simulink model "Simulink_Control_BlueROV_Modo_Deslizante"  (R2019a)
settings: Solver=VariableStepAuto  StartTime=0.0  StopTime=100*3  RelTol=1e-3
values from neighbouring files (symbols this model uses):
  a0 = 50    [Control_BlueROV_Modo_Deslizante.m]
  a1 = 1    [Control_BlueROV_Modo_Deslizante.m]
  B = 78.38    [Control_BlueROV_Modo_Deslizante.m]
  eta = 1    [Control_BlueROV_Modo_Deslizante.m]
  Ix = 0.16    [Control_BlueROV_Modo_Deslizante.m]
  Ixy = 0    [Control_BlueROV_Modo_Deslizante.m]
  Ixz = 0    [Control_BlueROV_Modo_Deslizante.m]
  Iy = 0.16    [Control_BlueROV_Modo_Deslizante.m]
  Iyz = 0    [Control_BlueROV_Modo_Deslizante.m]
  Iz = 0.16    [Control_BlueROV_Modo_Deslizante.m]
  Kp = -0.07    [Control_BlueROV_Modo_Deslizante.m]
  Kpdot = -0.12    [Control_BlueROV_Modo_Deslizante.m]
  Kpp = -1.55    [Control_BlueROV_Modo_Deslizante.m]
  m = 7.31    [Control_BlueROV_Modo_Deslizante.m]
  M = Mrb+Ma    [Control_BlueROV_Modo_Deslizante.m]
  Minv = inv(M)    [Control_BlueROV_Modo_Deslizante.m]
  Mq = -0.07    [Control_BlueROV_Modo_Deslizante.m]
  Mqdot = -0.12    [Control_BlueROV_Modo_Deslizante.m]
  Mqq = -1.55    [Control_BlueROV_Modo_Deslizante.m]
  Nr = -0.07    [Control_BlueROV_Modo_Deslizante.m]
  Nrdot = -0.12    [Control_BlueROV_Modo_Deslizante.m]
  Nrr = -1.55    [Control_BlueROV_Modo_Deslizante.m]
  W = 71.71    [Control_BlueROV_Modo_Deslizante.m]
  xb = 0    [Control_BlueROV_Modo_Deslizante.m]
  xg = 0    [Control_BlueROV_Modo_Deslizante.m]
  Xu = -4.03    [Control_BlueROV_Modo_Deslizante.m]
  Xudot = -5.5    [Control_BlueROV_Modo_Deslizante.m]
  Xuu = -18.18    [Control_BlueROV_Modo_Deslizante.m]
  yb = 0    [Control_BlueROV_Modo_Deslizante.m]
  yg = 0    [Control_BlueROV_Modo_Deslizante.m]
  Yv = -6.22    [Control_BlueROV_Modo_Deslizante.m]
  Yvdot = -12.7    [Control_BlueROV_Modo_Deslizante.m]
  Yvv = -21.66    [Control_BlueROV_Modo_Deslizante.m]
  zb = 0.00019    [Control_BlueROV_Modo_Deslizante.m]
  zg = 0    [Control_BlueROV_Modo_Deslizante.m]
  Zw = -5.18    [Control_BlueROV_Modo_Deslizante.m]
  Zwdot = -14.57    [Control_BlueROV_Modo_Deslizante.m]
  Zww = -36.99    [Control_BlueROV_Modo_Deslizante.m]
(part 1 of 2)
settings Model: Creator=andres lopez  LastModifiedBy=andres lopez

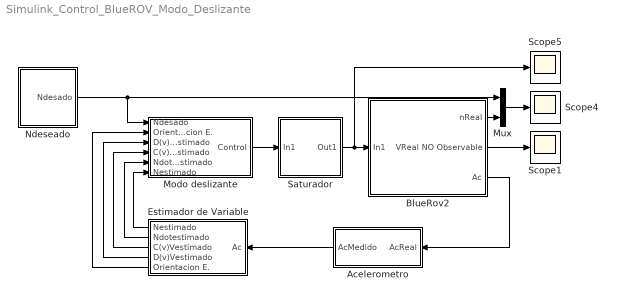
== system Simulink_Control_BlueROV_Modo_Deslizante ==
  Acelerometro : Subsystem
  BlueRov2 : Subsystem
  Estimador de Variable : Subsystem
  Modo deslizante : Subsystem
  Mux : Mux  Inputs=2
  Ndeseado : Subsystem
  Saturador : Subsystem
  Scope1 : Scope
  Scope4 : Scope
  Scope5 : Scope
  wires:
  BlueRov2/2("VReal NO Observable ") -> Scope1/1
  BlueRov2/1(nReal) -> Mux/2
  Ndeseado/1(Ndesado) -> Modo deslizante/1(Ndesado), Mux/1
  Mux/1 -> Scope4/1
  Saturador/1(Out1) -> Scope5/1, BlueRov2/1(In1)
  Modo deslizante/1(Control) -> Saturador/1(In1)
  Estimador de Variable/1(Nestimado) -> Modo deslizante/6(Nestimado)
  Estimador de Variable/2(Ndotestimado) -> Modo deslizante/5(Ndotestimado)
  Estimador de Variable/3(C(v)Vestimado) -> Modo deslizante/4(C(v)Vestimado)
  Estimador de Variable/4(D(v)Vestimado) -> Modo deslizante/3("D(v)Vestimado ")
  Estimador de Variable/5(Orientacion E.) -> Modo deslizante/2(Orientacion E.)
  BlueRov2/3(Ac) -> Acelerometro/1(AcReal)
  Acelerometro/1(AcMedido) -> Estimador de Variable/1(Ac)

== system Simulink_Control_BlueROV_Modo_Deslizante/Acelerometro ==
  AcReal : Inport
  Gain : Gain
  AcMedido : Outport
  wires:
  Gain/1 -> AcMedido/1
  AcReal/1 -> Gain/1

== system Simulink_Control_BlueROV_Modo_Deslizante/BlueRov2 ==
  In1 : Inport
  Add : Sum  Inputs=+---+
  C(v) : Subsystem
  D(v) : Subsystem
  Integrator : Integrator
  Integrator1 : Integrator
  J(n) : Subsystem
  "Perturbacion " : Step  Time=250  After=[2;-2;-3;0;0;0]  SampleTime=0
  g(n) : Subsystem
  inv(Matriz de masa Inercial) : Subsystem
  nReal : Outport
  "VReal NO Observable " : Outport  Port=2
  Ac : Outport  Port=3
  wires:
  In1/1 -> Add/1
  Add/1 -> inv(Matriz de masa Inercial)/1(Inercia)
  J(n)/1(Out1) -> Integrator1/1
  inv(Matriz de masa Inercial)/1(Aceleracion) -> Ac/1, Integrator/1
  g(n)/1(Out1) -> Add/2
  D(v)/1(Out1) -> Add/3
  Integrator1/1 -> g(n)/1(In1), J(n)/2(In2), nReal/1
  Integrator/1 -> "VReal NO Observable "/1, D(v)/1(In1), C(v)/1(In1), J(n)/1(In1)
  C(v)/1(Out1) -> Add/4
  "Perturbacion "/1 -> Add/5

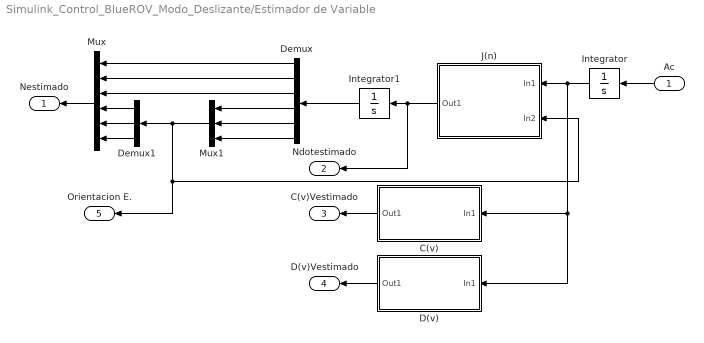
== system Simulink_Control_BlueROV_Modo_Deslizante/Estimador de Variable ==
  Ac : Inport
  C(v) : Subsystem
  D(v) : Subsystem
  Demux : Demux  Outputs=6
  Demux1 : Demux  Outputs=3
  Integrator : Integrator
  Integrator1 : Integrator
  J(n) : Subsystem
  Mux : Mux  Inputs=6
  Mux1 : Mux  Inputs=3
  Nestimado : Outport
  Ndotestimado : Outport  Port=2
  C(v)Vestimado : Outport  Port=3
  D(v)Vestimado : Outport  Port=4
  Orientacion E. : Outport  Port=5
  wires:
  Ac/1 -> Integrator/1
  Integrator/1 -> D(v)/1(In1), C(v)/1(In1), J(n)/1(In1)
  J(n)/1(Out1) -> Ndotestimado/1, Integrator1/1
  C(v)/1(Out1) -> C(v)Vestimado/1
  D(v)/1(Out1) -> D(v)Vestimado/1
  Integrator1/1 -> Demux/1
  Demux/1 -> Mux/1
  Demux/2 -> Mux/2
  Demux1/2 -> Mux/5
  Demux1/1 -> Mux/4
  Demux1/3 -> Mux/6
  Mux/1 -> Nestimado/1
  Demux/3 -> Mux/3
  Mux1/1 -> Orientacion E./1, J(n)/2(In2), Demux1/1
  Demux/4 -> Mux1/1
  Demux/5 -> Mux1/2
  Demux/6 -> Mux1/3

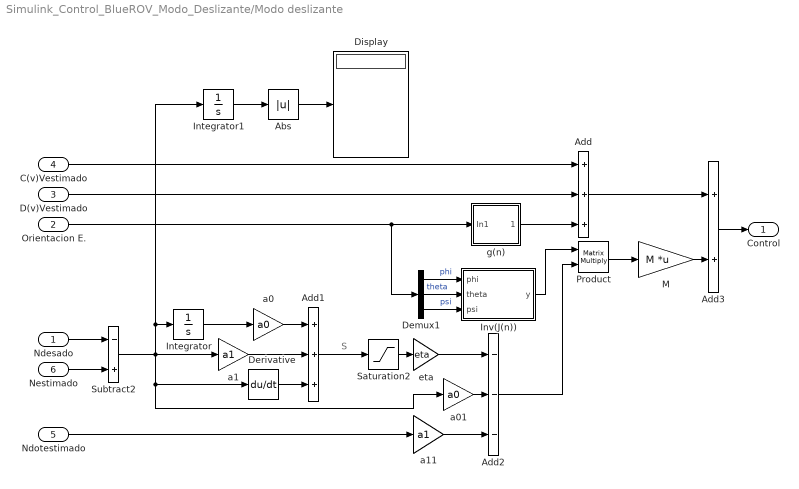
== system Simulink_Control_BlueROV_Modo_Deslizante/Modo deslizante ==
  note: S
  Ndesado : Inport
  Orientacion E. : Inport  Port=2
  "D(v)Vestimado " : Inport  Port=3
  C(v)Vestimado : Inport  Port=4
  Ndotestimado : Inport  Port=5
  Nestimado : Inport  Port=6
  Abs : Abs
  Add : Sum  Inputs=+++
  Add1 : Sum  Inputs=+++
  Add2 : Sum  Inputs=---
  Add3 : Sum
  Demux1 : Demux  Outputs=3
  Derivative : Derivative
  Display : Display
  Integrator : Integrator
  Integrator1 : Integrator
  Inv(J(n)) : MATLAB Function  TreatAsAtomicUnit=on
  M : Gain  Gain=M  Multiplication=Matrix(K*u) (u vector)
  Product : Product  Multiplication=Matrix(*)
  Saturation2 : Saturate  UpperLimit=1  LowerLimit=-1
  Subtract2 : Sum  Inputs=-+
  "a0 " : Gain  Gain=a0
  a01 : Gain  Gain=a0
  a1 : Gain  Gain=a1
  a11 : Gain  Gain=a1
  eta : Gain  Gain=eta
  g(n) : Subsystem
  Control : Outport
  wires:
  Ndotestimado/1 -> a11/1
  Orientacion E./1 -> Demux1/1, g(n)/1(In1)
  a11/1 -> Add2/3
  eta/1 -> Add2/1
  Demux1/1 -> Inv(J(n))/1(phi)  "phi"
  Demux1/3 -> Inv(J(n))/3(psi)  "psi"
  Add2/1 -> Product/2
  Saturation2/1 -> eta/1
  Product/1 -> M/1
  Inv(J(n))/1(y) -> Product/1
  a01/1 -> Add2/2
  Demux1/2 -> Inv(J(n))/2(theta)  "theta"
  Integrator1/1 -> Abs/1
  Abs/1 -> Display/1
  Add3/1 -> Control/1
  M/1 -> Add3/2
  Add/1 -> Add3/1
  Nestimado/1 -> Subtract2/2
  Ndesado/1 -> Subtract2/1
  g(n)/1(Out1) -> Add/3
  "D(v)Vestimado "/1 -> Add/2
  C(v)Vestimado/1 -> Add/1
  Subtract2/1 -> Integrator1/1, Integrator/1, a1/1, Derivative/1, a01/1
  Add1/1 -> Saturation2/1
  Derivative/1 -> Add1/3
  "a0 "/1 -> Add1/1
  a1/1 -> Add1/2
  Integrator/1 -> "a0 "/1

== system Simulink_Control_BlueROV_Modo_Deslizante/Ndeseado ==
  Euler 1 : Constant  Value=[0;0;0]
  Mux2 : Mux
  Uniform Random Number4 : UniformRandomNumber  Minimum=-10  Maximum=10  Seed=2  SampleTime=100
  Uniform Random Number5 : UniformRandomNumber  Minimum=0  Maximum=10  Seed=1  SampleTime=100
  Uniform Random Number6 : UniformRandomNumber  Minimum=-10  Maximum=10  Seed=3  SampleTime=100
  Ndesado : Outport
  wires:
  Uniform Random Number4/1 -> Mux2/2
  Uniform Random Number5/1 -> Mux2/3
  Euler 1/1 -> Mux2/4
  Mux2/1 -> Ndesado/1
  Uniform Random Number6/1 -> Mux2/1

== system Simulink_Control_BlueROV_Modo_Deslizante/Saturador ==
  In1 : Inport
  Demux3 : Demux  Outputs=6
  Mux1 : Mux  Inputs=3
  Mux2 : Mux
  Saturation : Saturate  UpperLimit=6.5  LowerLimit=-6.5
  Saturation1 : Saturate  UpperLimit=7.5  LowerLimit=-7.5
  Saturation2 : Saturate  UpperLimit=11  LowerLimit=4
  Saturation3 : Saturate  UpperLimit=3  LowerLimit=-3
  Out1 : Outport
  wires:
  Demux3/1 -> Saturation/1
  Saturation2/1 -> Mux2/3
  Saturation/1 -> Mux2/1
  Saturation3/1 -> Mux2/4
  Saturation1/1 -> Mux2/2
  Demux3/3 -> Saturation2/1
  Mux1/1 -> Saturation3/1
  Demux3/6 -> Mux1/3
  Demux3/2 -> Saturation1/1
  Demux3/5 -> Mux1/2
  Demux3/4 -> Mux1/1
  Mux2/1 -> Out1/1
  In1/1 -> Demux3/1

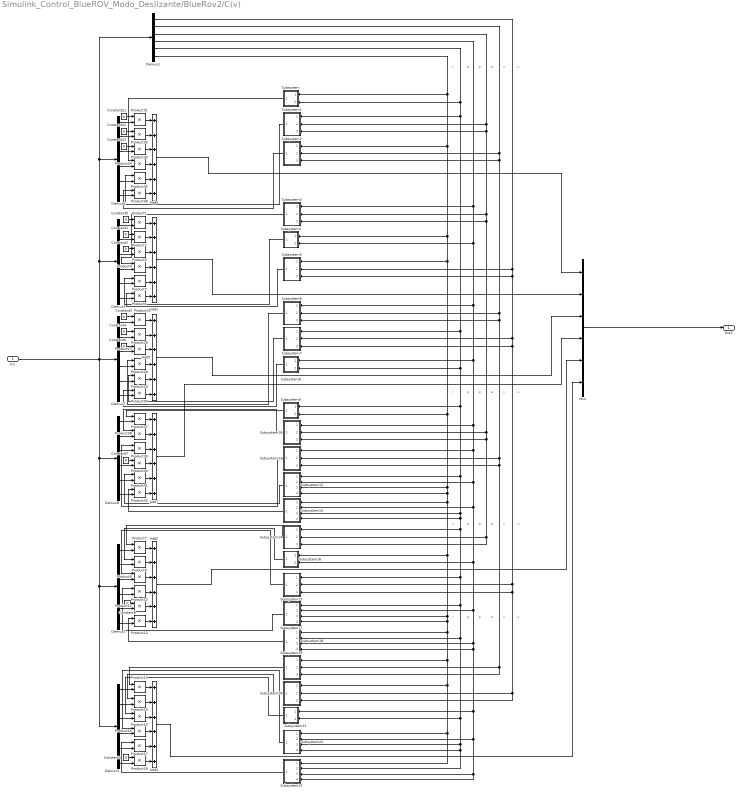
== system Simulink_Control_BlueROV_Modo_Deslizante/BlueRov2/C(v) ==
  note: u
  note: v
  note: w
  note: p
  note: q
  note: r
  note: v
  note: p
  note: u
  note: w
  note: q
  note: r
  note: v
  note: r
  note: w
  note: u
  note: q
  note: p
  note: v
  note: r
  note: w
  note: u
  note: q
  note: p
  In1 : Inport
  Add{1..3,5..7} (6 alike) : Sum  Inputs=++++++
  Constant{1..9,21..23} (12 alike) : Constant  Value=0
  Demux{1..3,5..8} (7 alike) : Demux  Outputs=6
  Mux : Mux  Inputs=6
  Product{1..18,25..42} (36 alike) : Product
  Subsystem : Subsystem
  Subsystem1 : Subsystem
  Subsystem10 : Subsystem
  Subsystem11 : Subsystem
  Subsystem12 : Subsystem
  Subsystem13 : Subsystem
  Subsystem14 : Subsystem
  Subsystem15 : Subsystem
  Subsystem16 : Subsystem
  Subsystem17 : Subsystem
  Subsystem18 : Subsystem
  Subsystem19 : Subsystem
  Subsystem2 : Subsystem
  Subsystem20 : Subsystem
  Subsystem21 : Subsystem
  Subsystem22 : Subsystem
  Subsystem23 : Subsystem
  Subsystem3 : Subsystem
  Subsystem4 : Subsystem
  Subsystem5 : Subsystem
  Subsystem6 : Subsystem
  Subsystem7 : Subsystem
  Subsystem8 : Subsystem
  Subsystem9 : Subsystem
  Out1 : Outport
  wires:
  In1/1 -> Demux5/1, Demux6/1, Demux1/1, Demux7/1, Demux8/1, Demux3/1, Demux2/1
  Product39/1 -> Add7/3
  Demux8/2 -> Product38/2
  Product36/1 -> Add6/6
  Product31/1 -> Add6/1
  Product35/1 -> Add6/5
  Demux6/2 -> Product32/2
  Demux6/4 -> Product34/2
  Demux6/5 -> Product35/2
  Product33/1 -> Add6/3
  Demux6/3 -> Product33/2
  Product5/1 -> Add1/5
  Demux5/2 -> Product2/2
  Product32/1 -> Add6/2
  Product41/1 -> Add7/5
  Product34/1 -> Add6/4
  Product2/1 -> Add1/2
  Demux8/5 -> Product41/2
  Product1/1 -> Add1/1
  Product18/1 -> Add3/6
  Product3/1 -> Add1/3
  Demux8/3 -> Product39/2
  Product8/1 -> Add2/2
  Demux2/6 -> Product12/2
  Product4/1 -> Add1/4
  Product37/1 -> Add7/1
  Demux5/1 -> Product1/2
  Demux8/6 -> Product42/2
  Demux5/4 -> Product4/2
  Demux5/5 -> Product5/2
  Product17/1 -> Add3/5
  Demux5/3 -> Product3/2
  Demux6/1 -> Product31/2
  Product13/1 -> Add3/1
  Product14/1 -> Add3/2
  Product40/1 -> Add7/4
  Product15/1 -> Add3/3
  Demux8/4 -> Product40/2
  Demux7/2 -> Product26/2
  Product42/1 -> Add7/6
  Product12/1 -> Add2/6
  Product26/1 -> Add5/2
  Product6/1 -> Add1/6
  Demux6/6 -> Product36/2
  Demux5/6 -> Product6/2
  Product29/1 -> Add5/5
  Product28/1 -> Add5/4
  Demux7/3 -> Product27/2
  Product16/1 -> Add3/4
  Product10/1 -> Add2/4
  Demux7/5 -> Product29/2
  Product9/1 -> Add2/3
  Product38/1 -> Add7/2
  Demux2/4 -> Product10/2
  Demux2/2 -> Product8/2
  Demux8/1 -> Product37/2
  Demux2/5 -> Product11/2
  Product7/1 -> Add2/1
  Product11/1 -> Add2/5
  Mux/1 -> Out1/1
  Demux7/4 -> Product28/2
  Demux2/1 -> Product7/2
  Demux7/6 -> Product30/2
  Product25/1 -> Add5/1
  Product27/1 -> Add5/3
  Product30/1 -> Add5/6
  Demux7/1 -> Product25/2
  Demux2/3 -> Product9/2
  Constant21/1 -> Product31/1
  Constant22/1 -> Product32/1
  Constant23/1 -> Product33/1
  Demux3/6 -> Product18/2
  Demux3/5 -> Product17/2
  Demux3/4 -> Product16/2
  Demux3/3 -> Product15/2
  Demux3/2 -> Product14/2
  Demux3/1 -> Product13/2
  Constant5/1 -> Product1/1
  Constant1/1 -> Product2/1
  Constant2/1 -> Product3/1
  Constant3/1 -> Product25/1
  Constant4/1 -> Product26/1
  Constant6/1 -> Product27/1
  Constant7/1 -> Product40/1
  Constant8/1 -> Product11/1
  Constant9/1 -> Product18/1
  Demux1/1 -> Subsystem5/2(In2), Subsystem15/2(In2), Subsystem15/3(In3), Subsystem20/2(In2), Subsystem20/3(In3), Subsystem7/3(In3), Subsystem7/2(In2), Subsystem5/3(In3)
  Demux1/2 -> Subsystem11/3(In3), Subsystem19/2(In2), Subsystem19/3(In3), Subsystem11/2(In2), Subsystem6/3(In3), Subsystem6/2(In2), Subsystem2/3(In3), Subsystem2/2(In2)
  Demux1/3 -> Subsystem3/2(In2), Subsystem3/3(In3), Subsystem10/2(In2), Subsystem10/3(In3), Subsystem14/2(In2), Subsystem14/3(In3), Subsystem1/3(In3), Subsystem1/2(In2)
  Subsystem/1(Out1) -> Product34/1
  Subsystem1/1(Out1) -> Product35/1
  Subsystem2/1(Out1) -> Product36/1
  Add6/1 -> Mux/1
  Subsystem3/1(Out1) -> Product4/1
  Subsystem4/1(Out1) -> Product5/1
  Subsystem5/1(Out1) -> Product6/1
  Add1/1 -> Mux/2
  Subsystem6/1(Out1) -> Product28/1
  Subsystem7/1(Out1) -> Product29/1
  Subsystem8/1(Out1) -> Product30/1
  Add5/1 -> Mux/3
  Subsystem9/1(Out1) -> Product37/1
  Subsystem10/1(Out1) -> Product38/1
  Subsystem11/1(Out1) -> Product39/1
  Subsystem12/1(Out1) -> Product41/1
  Subsystem13/1(Out1) -> Product42/1
  Add7/1 -> Mux/4
  Subsystem14/1(Out1) -> Product7/1
  Demux1/4 -> Subsystem3/1(In1), Subsystem4/2(In2), Subsystem8/1(In1), Subsystem10/1(In1), Subsystem11/1(In1), Subsystem12/2(In2), Subsystem13/2(In2), Subsystem16/2(In2), Subsystem17/2(In2), Subsystem18/3(In3), Subsystem18/4(In4), Subsystem21/1(In1), Subsystem22/2(In2), Subsystem23/3(In3), Subsystem23/4(In4), Subsystem6/1(In1)
  Subsystem16/1(Out1) -> Product8/1
  Subsystem15/1(Out1) -> Product9/1
  Demux1/6 -> Subsystem4/1(In1), Subsystem5/1(In1), Subsystem12/4(In4), Subsystem13/1(In1), Subsystem16/1(In1), Subsystem17/4(In4), Subsystem18/1(In1), Subsystem19/1(In1), Subsystem20/1(In1), Subsystem22/1(In1), Subsystem23/1(In1), Subsystem17/3(In3), Subsystem12/3(In3), Subsystem9/2(In2), Subsystem2/1(In1), Subsystem/1(In1)
  Subsystem17/1(Out1) -> Product10/1
  Subsystem18/1(Out1) -> Product12/1
  Subsystem19/1(Out1) -> Product13/1
  Add2/1 -> Mux/5
  Subsystem20/1(Out1) -> Product14/1
  Subsystem21/1(Out1) -> Product15/1
  Demux1/5 -> Subsystem12/1(In1), Subsystem13/3(In3), Subsystem13/4(In4), Subsystem15/1(In1), Subsystem17/1(In1), Subsystem18/2(In2), Subsystem21/2(In2), Subsystem22/4(In4), Subsystem23/2(In2), Subsystem22/3(In3), Subsystem14/1(In1), Subsystem9/1(In1), Subsystem8/2(In2), Subsystem7/1(In1), Subsystem1/1(In1), Subsystem/2(In2)
  Subsystem22/1(Out1) -> Product16/1
  Subsystem23/1(Out1) -> Product17/1
  Add3/1 -> Mux/6

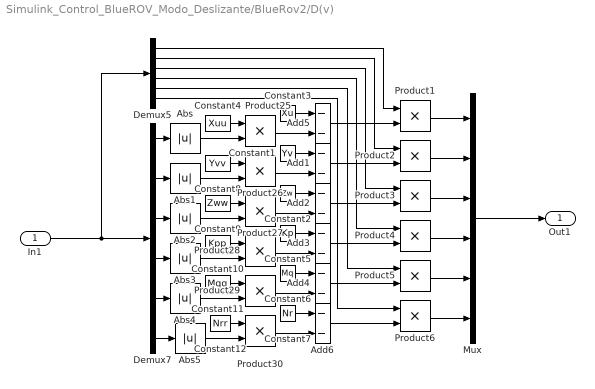
== system Simulink_Control_BlueROV_Modo_Deslizante/BlueRov2/D(v) ==
  In1 : Inport
  Abs{,1..5} (6 alike) : Abs
  Add{1..6} (6 alike) : Sum  Inputs=--
  Constant1 : Constant  Value=Yv
  Constant10 : Constant  Value=Kpp
  Constant11 : Constant  Value=Mqq
  Constant12 : Constant  Value=Nrr
  Constant2 : Constant  Value=Zw
  Constant3 : Constant  Value=Xu
  Constant4 : Constant  Value=Xuu
  Constant5 : Constant  Value=Kp
  Constant6 : Constant  Value=Mq
  Constant7 : Constant  Value=Nr
  Constant8 : Constant  Value=Yvv
  Constant9 : Constant  Value=Zww
  Demux5 : Demux  Outputs=6
  Demux7 : Demux  Outputs=6
  Mux : Mux  Inputs=6
  Product{1..6,25..30} (12 alike) : Product
  Out1 : Outport
  wires:
  In1/1 -> Demux5/1, Demux7/1
  ? -> ?
  ? -> ?
  Mux/1 -> Out1/1
  Abs/1 -> Product25/2
  Demux7/2 -> Abs1/1
  Abs1/1 -> Product26/2
  Demux7/1 -> Abs/1
  Demux7/3 -> Abs2/1
  Abs2/1 -> Product27/2
  Demux7/4 -> Abs3/1
  Abs3/1 -> Product28/2
  Abs4/1 -> Product29/2
  Demux7/5 -> Abs4/1
  Abs5/1 -> Product30/2
  Demux7/6 -> Abs5/1
  Product25/1 -> Add5/2
  Product26/1 -> Add1/2
  Product27/1 -> Add2/2
  Product28/1 -> Add3/2
  Product29/1 -> Add4/2
  Product30/1 -> Add6/2
  Product6/1 -> Mux/6
  Product5/1 -> Mux/5
  Product4/1 -> Mux/4
  Product3/1 -> Mux/3
  Product2/1 -> Mux/2
  Product1/1 -> Mux/1
  Add6/1 -> Product6/2
  Add4/1 -> Product5/2
  Add3/1 -> Product4/2
  Add2/1 -> Product3/2
  Add1/1 -> Product2/2
  Add5/1 -> Product1/2
  Demux5/6 -> Product6/1
  Demux5/5 -> Product5/1
  Demux5/4 -> Product4/1
  Demux5/3 -> Product3/1
  Demux5/2 -> Product2/1
  Demux5/1 -> Product1/1
  Constant1/1 -> Add1/1
  Constant2/1 -> Add2/1
  Constant3/1 -> Add5/1
  Constant5/1 -> Add3/1
  Constant6/1 -> Add4/1
  Constant7/1 -> Add6/1
  Constant4/1 -> Product25/1
  Constant8/1 -> Product26/1
  Constant12/1 -> Product30/1
  Constant11/1 -> Product29/1
  Constant10/1 -> Product28/1
  Constant9/1 -> Product27/1

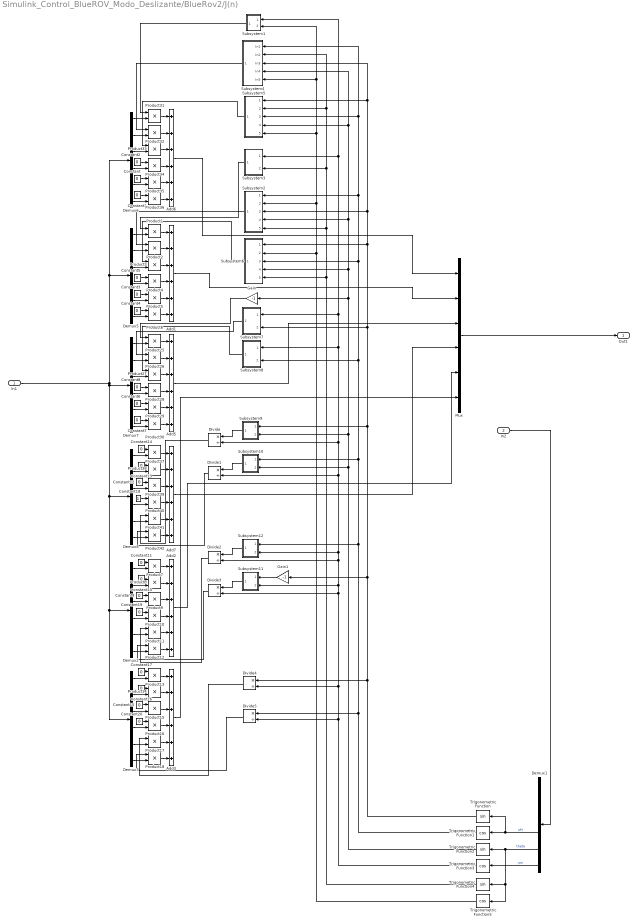
== system Simulink_Control_BlueROV_Modo_Deslizante/BlueRov2/J(n) ==
  In1 : Inport
  In2 : Inport  Port=2
  Add{1..3,5..7} (6 alike) : Sum  Inputs=++++++
  Constant{,1..17,19..20} (20 alike) : Constant  Value=0
  Constant18 : Constant
  Demux{1..3,5..8} (7 alike) : Demux  Outputs=6
  Divide{,1..5} (6 alike) : Product  Inputs=*/
  Gain : Gain  Gain=-1
  Gain1 : Gain  Gain=-1
  Mux : Mux  Inputs=6
  Product{1..18,25..42} (36 alike) : Product
  Subsystem1 : Subsystem
  Subsystem10 : Subsystem
  Subsystem11 : Subsystem
  Subsystem12 : Subsystem
  Subsystem2 : Subsystem
  Subsystem3 : Subsystem
  Subsystem4 : Subsystem
  Subsystem5 : Subsystem
  Subsystem6 : Subsystem
  Subsystem7 : Subsystem
  Subsystem8 : Subsystem
  Subsystem9 : Subsystem
  Trigonometric Function : Trigonometry
  Trigonometric Function1 : Trigonometry  Operator=cos
  Trigonometric Function2 : Trigonometry
  Trigonometric Function3 : Trigonometry  Operator=cos
  Trigonometric Function4 : Trigonometry
  Trigonometric Function5 : Trigonometry  Operator=cos
  Out1 : Outport
  wires:
  Divide5/1 -> Product18/1
  Divide3/1 -> Product12/1
  Subsystem1/1(Out1) -> Product31/1
  Constant12/1 -> Product39/1
  Subsystem5/1(Out1) -> Product33/1
  Constant13/1 -> Product38/1
  Subsystem10/1(Out1) -> Divide1/1
  Divide1/1 -> Product42/1
  Demux7/3 -> Product27/2
  Product28/1 -> Add5/4
  Product29/1 -> Add5/5
  Product25/1 -> Add5/1
  Product30/1 -> Add5/6
  Demux7/6 -> Product30/2
  Constant8/1 -> Product28/1
  Demux7/1 -> Product25/2
  Demux7/4 -> Product28/2
  Product27/1 -> Add5/3
  Constant6/1 -> Product29/1
  Product11/1 -> Add2/5
  Demux2/3 -> Product9/2
  Product7/1 -> Add2/1
  Demux2/1 -> Product7/2
  Demux2/5 -> Product11/2
  Demux2/4 -> Product10/2
  Product9/1 -> Add2/3
  Demux2/2 -> Product8/2
  Constant10/1 -> Product8/1
  Trigonometric Function3/1 -> Divide5/2, Divide4/2, Divide3/2, Subsystem11/2(In2), Divide2/2, Subsystem12/2(In2), Divide1/2, Divide/2, Subsystem8/1(In1), Subsystem7/1(In1), Subsystem3/1(In1), Subsystem1/1(In1)
  Demux8/2 -> Product38/2
  Product39/1 -> Add7/3
  Product38/1 -> Add7/2
  In1/1 -> Demux7/1, Demux8/1, Demux3/1, Demux2/1, Demux5/1, Demux6/1
  Subsystem9/1(Out1) -> Divide/1
  Add2/1 -> Mux/5
  Subsystem11/1(Out1) -> Divide3/1
  Product10/1 -> Add2/4
  Subsystem12/1(Out1) -> Divide2/1
  Constant19/1 -> Product10/1
  Trigonometric Function1/1 -> Divide5/1, Subsystem10/1(In1), Subsystem8/2(In2), Subsystem6/3(In3), Subsystem2/1(In1), Subsystem5/3(In3), Subsystem4/1(In1), Subsystem12/1(In1)
  Add1/1 -> Mux/2
  Mux/1 -> Out1/1
  Add6/1 -> Mux/1
  Add3/1 -> Mux/6
  Product12/1 -> Add2/6
  Add7/1 -> Mux/4
  Divide4/1 -> Product17/1
  Add5/1 -> Mux/3
  Product26/1 -> Add5/2
  Constant7/1 -> Product30/1
  Trigonometric Function/1 -> Divide4/1, Gain1/1, Subsystem9/1(In1), Subsystem7/2(In2), Subsystem6/1(In1), Subsystem2/3(In3), Subsystem5/1(In1), Subsystem4/3(In3)
  Constant14/1 -> Product37/1
  Gain/1 -> Product25/1
  Trigonometric Function5/1 -> Subsystem6/2(In2), Subsystem5/5(In5), Subsystem4/5(In5), Subsystem1/2(In2), Subsystem2/2(In2)
  Subsystem8/1(Out1) -> Product27/1
  Subsystem3/1(Out1) -> Product1/1
  Subsystem6/1(Out1) -> Product3/1
  Demux7/2 -> Product26/2
  Constant20/1 -> Product16/1
  Subsystem7/1(Out1) -> Product26/1
  Demux7/5 -> Product29/2
  Constant15/1 -> Product15/1
  Constant16/1 -> Product14/1
  Demux3/2 -> Product14/2
  Product15/1 -> Add3/3
  Constant17/1 -> Product13/1
  Product14/1 -> Add3/2
  Constant11/1 -> Product7/1
  Trigonometric Function4/1 -> Subsystem6/5(In5), Subsystem2/5(In5), Subsystem3/2(In2), Subsystem5/2(In2), Subsystem4/2(In2)
  Subsystem4/1(Out1) -> Product32/1
  Product13/1 -> Add3/1
  Product16/1 -> Add3/4
  Demux3/1 -> Product13/2
  Demux3/4 -> Product16/2
  Demux3/3 -> Product15/2
  Trigonometric Function2/1 -> Subsystem10/2(In2), Subsystem9/2(In2), Gain/1, Subsystem6/4(In4), Subsystem2/4(In4), Subsystem5/4(In4), Subsystem4/4(In4)
  Constant1/1 -> Product36/1
  Product17/1 -> Add3/5
  Demux5/3 -> Product3/2
  Product6/1 -> Add1/6
  Demux5/5 -> Product5/2
  Demux5/4 -> Product4/2
  Demux5/1 -> Product1/2
  Demux1/4 -> Trigonometric Function/1, Trigonometric Function1/1  "phi"
  Constant4/1 -> Product6/1
  Constant2/1 -> Product34/1
  Constant/1 -> Product35/1
  Demux8/6 -> Product42/2
  Demux3/5 -> Product17/2
  Product4/1 -> Add1/4
  Constant18/1 -> Product40/1
  Product37/1 -> Add7/1
  Demux2/6 -> Product12/2
  Demux8/4 -> Product40/2
  Gain1/1 -> Subsystem11/1(In1)
  Product42/1 -> Add7/6
  Constant3/1 -> Product5/1
  Product8/1 -> Add2/2
  Demux8/5 -> Product41/2
  Product1/1 -> Add1/1
  Demux8/3 -> Product39/2
  Product3/1 -> Add1/3
  Divide2/1 -> Product11/1
  Product18/1 -> Add3/6
  Demux1/6 -> Trigonometric Function5/1, Trigonometric Function4/1  "psi"
  Constant5/1 -> Product4/1
  Demux5/2 -> Product2/2
  Divide/1 -> Product41/1
  Product32/1 -> Add6/2
  Product2/1 -> Add1/2
  Product34/1 -> Add6/4
  Demux6/1 -> Product31/2
  Demux6/6 -> Product36/2
  Product41/1 -> Add7/5
  Demux6/5 -> Product35/2
  Product5/1 -> Add1/5
  Constant9/1 -> Product9/1
  Demux3/6 -> Product18/2
  Product33/1 -> Add6/3
  Demux1/5 -> Trigonometric Function3/1, Trigonometric Function2/1  "theta"
  Demux6/4 -> Product34/2
  Demux6/3 -> Product33/2
  Demux5/6 -> Product6/2
  Product36/1 -> Add6/6
  Demux6/2 -> Product32/2
  Subsystem2/1(Out1) -> Product2/1
  Product40/1 -> Add7/4
  Demux8/1 -> Product37/2
  Product31/1 -> Add6/1
  Product35/1 -> Add6/5
  In2/1 -> Demux1/1

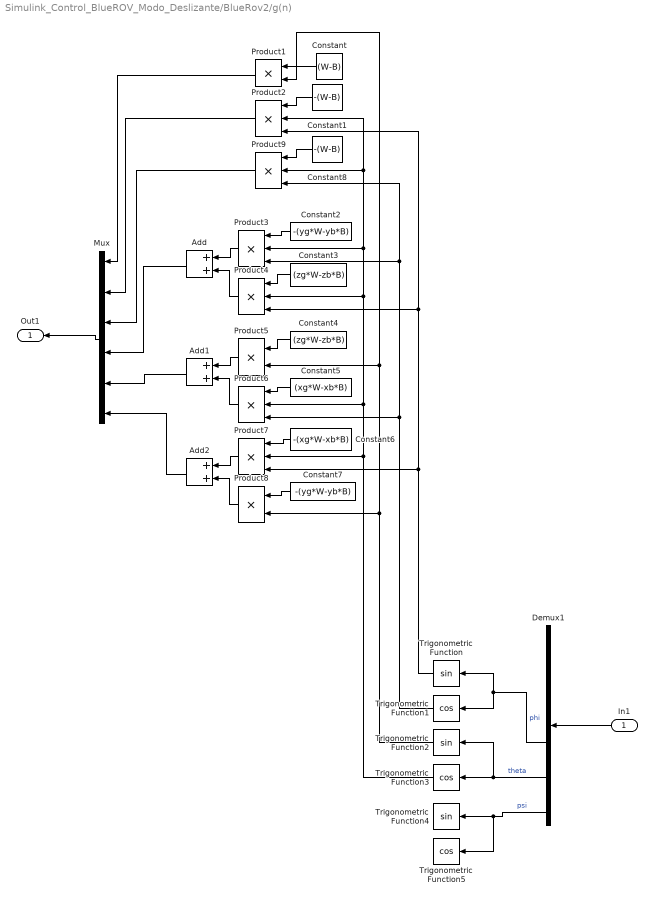
== system Simulink_Control_BlueROV_Modo_Deslizante/BlueRov2/g(n) ==
  In1 : Inport
  Add : Sum
  Add1 : Sum
  Add2 : Sum
  Constant : Constant  Value=(W-B)
  Constant1 : Constant  Value=-(W-B)
  Constant2 : Constant  Value=-(yg*W-yb*B)
  Constant3 : Constant  Value=(zg*W-zb*B)
  Constant4 : Constant  Value=(zg*W-zb*B)
  Constant5 : Constant  Value=(xg*W-xb*B)
  Constant6 : Constant  Value=-(xg*W-xb*B)
  Constant7 : Constant  Value=-(yg*W-yb*B)
  Constant8 : Constant  Value=-(W-B)
  Demux1 : Demux  Outputs=6
  Mux : Mux  Inputs=6
  Product1 : Product
  Product{2..4,6..7,9} (6 alike) : Product  Inputs=3
  Product5 : Product
  Product8 : Product
  Trigonometric Function : Trigonometry
  Trigonometric Function1 : Trigonometry  Operator=cos
  Trigonometric Function2 : Trigonometry
  Trigonometric Function3 : Trigonometry  Operator=cos
  Trigonometric Function4 : Trigonometry
  Trigonometric Function5 : Trigonometry  Operator=cos
  Out1 : Outport
  wires:
  Demux1/6 -> Trigonometric Function5/1, Trigonometric Function4/1  "psi"
  Demux1/4 -> Trigonometric Function/1, Trigonometric Function1/1  "phi"
  Demux1/5 -> Trigonometric Function2/1, Trigonometric Function3/1  "theta"
  In1/1 -> Demux1/1
  Mux/1 -> Out1/1
  Product1/1 -> Mux/1
  Constant/1 -> Product1/1
  Trigonometric Function2/1 -> Product8/2, Product5/2, Product1/2
  Constant1/1 -> Product2/1
  Trigonometric Function/1 -> Product7/3, Product4/3, Product2/3
  Product2/1 -> Mux/2
  Product7/1 -> Add2/1
  Product8/1 -> Add2/2
  Product6/1 -> Add1/2
  Constant5/1 -> Product6/1
  Constant2/1 -> Product3/1
  Constant4/1 -> Product5/1
  Product4/1 -> Add/2
  Constant3/1 -> Product4/1
  Product3/1 -> Add/1
  Product5/1 -> Add1/1
  Constant7/1 -> Product8/1
  Constant8/1 -> Product9/1
  Product9/1 -> Mux/3
  Add/1 -> Mux/4
  Add1/1 -> Mux/5
  Constant6/1 -> Product7/1
  Add2/1 -> Mux/6
  Trigonometric Function1/1 -> Product6/3, Product3/3, Product9/3
  Trigonometric Function3/1 -> Product7/2, Product6/2, Product4/2, Product3/2, Product9/2, Product2/2

== system Simulink_Control_BlueROV_Modo_Deslizante/BlueRov2/inv(Matriz de masa Inercial) ==
  Inercia : Inport
  INVM : Gain  Gain=Minv  Multiplication=Matrix(K*u) (u vector)
  Aceleracion : Outport
  wires:
  INVM/1 -> Aceleracion/1
  Inercia/1 -> INVM/1

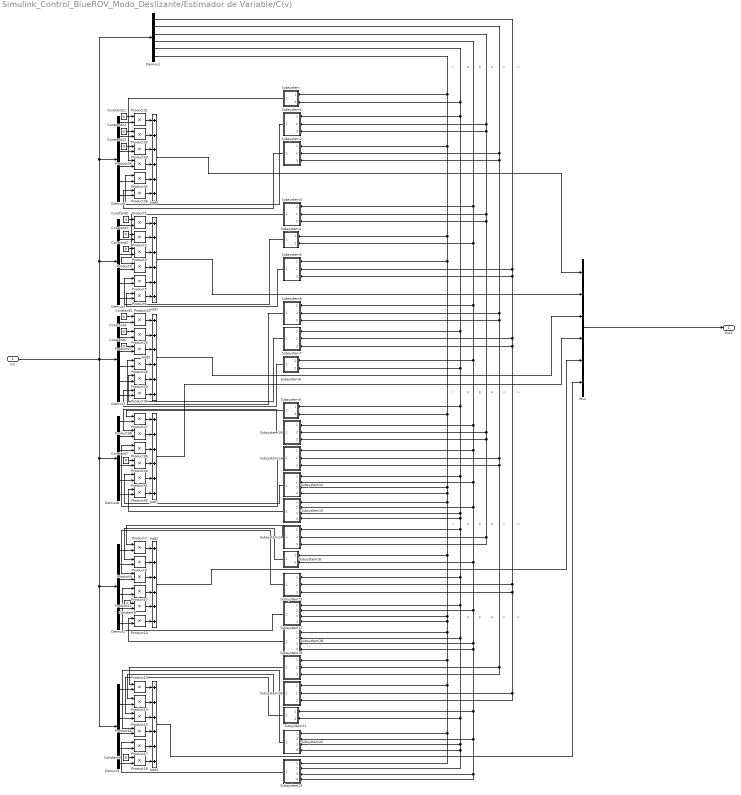
== system Simulink_Control_BlueROV_Modo_Deslizante/Estimador de Variable/C(v) ==
  note: u
  note: v
  note: w
  note: p
  note: q
  note: r
  note: v
  note: p
  note: u
  note: w
  note: q
  note: r
  note: v
  note: r
  note: w
  note: u
  note: q
  note: p
  note: v
  note: r
  note: w
  note: u
  note: q
  note: p
  In1 : Inport
  Add{1..3,5..7} (6 alike) : Sum  Inputs=++++++
  Constant{1..9,21..23} (12 alike) : Constant  Value=0
  Demux{1..3,5..8} (7 alike) : Demux  Outputs=6
  Mux : Mux  Inputs=6
  Product{1..18,25..42} (36 alike) : Product
  Subsystem : Subsystem
  Subsystem1 : Subsystem
  Subsystem10 : Subsystem
  Subsystem11 : Subsystem
  Subsystem12 : Subsystem
  Subsystem13 : Subsystem
  Subsystem14 : Subsystem
  Subsystem15 : Subsystem
  Subsystem16 : Subsystem
  Subsystem17 : Subsystem
  Subsystem18 : Subsystem
  Subsystem19 : Subsystem
  Subsystem2 : Subsystem
  Subsystem20 : Subsystem
  Subsystem21 : Subsystem
  Subsystem22 : Subsystem
  Subsystem23 : Subsystem
  Subsystem3 : Subsystem
  Subsystem4 : Subsystem
  Subsystem5 : Subsystem
  Subsystem6 : Subsystem
  Subsystem7 : Subsystem
  Subsystem8 : Subsystem
  Subsystem9 : Subsystem
  Out1 : Outport
  wires:
  In1/1 -> Demux5/1, Demux6/1, Demux1/1, Demux7/1, Demux8/1, Demux3/1, Demux2/1
  Product39/1 -> Add7/3
  Demux8/2 -> Product38/2
  Product36/1 -> Add6/6
  Product31/1 -> Add6/1
  Product35/1 -> Add6/5
  Demux6/2 -> Product32/2
  Demux6/4 -> Product34/2
  Demux6/5 -> Product35/2
  Product33/1 -> Add6/3
  Demux6/3 -> Product33/2
  Product5/1 -> Add1/5
  Demux5/2 -> Product2/2
  Product32/1 -> Add6/2
  Product41/1 -> Add7/5
  Product34/1 -> Add6/4
  Product2/1 -> Add1/2
  Demux8/5 -> Product41/2
  Product1/1 -> Add1/1
  Product18/1 -> Add3/6
  Product3/1 -> Add1/3
  Demux8/3 -> Product39/2
  Product8/1 -> Add2/2
  Demux2/6 -> Product12/2
  Product4/1 -> Add1/4
  Product37/1 -> Add7/1
  Demux5/1 -> Product1/2
  Demux8/6 -> Product42/2
  Demux5/4 -> Product4/2
  Demux5/5 -> Product5/2
  Product17/1 -> Add3/5
  Demux5/3 -> Product3/2
  Demux6/1 -> Product31/2
  Product13/1 -> Add3/1
  Product14/1 -> Add3/2
  Product40/1 -> Add7/4
  Product15/1 -> Add3/3
  Demux8/4 -> Product40/2
  Demux7/2 -> Product26/2
  Product42/1 -> Add7/6
  Product12/1 -> Add2/6
  Product26/1 -> Add5/2
  Product6/1 -> Add1/6
  Demux6/6 -> Product36/2
  Demux5/6 -> Product6/2
  Product29/1 -> Add5/5
  Product28/1 -> Add5/4
  Demux7/3 -> Product27/2
  Product16/1 -> Add3/4
  Product10/1 -> Add2/4
  Demux7/5 -> Product29/2
  Product9/1 -> Add2/3
  Product38/1 -> Add7/2
  Demux2/4 -> Product10/2
  Demux2/2 -> Product8/2
  Demux8/1 -> Product37/2
  Demux2/5 -> Product11/2
  Product7/1 -> Add2/1
  Product11/1 -> Add2/5
  Mux/1 -> Out1/1
  Demux7/4 -> Product28/2
  Demux2/1 -> Product7/2
  Demux7/6 -> Product30/2
  Product25/1 -> Add5/1
  Product27/1 -> Add5/3
  Product30/1 -> Add5/6
  Demux7/1 -> Product25/2
  Demux2/3 -> Product9/2
  Constant21/1 -> Product31/1
  Constant22/1 -> Product32/1
  Constant23/1 -> Product33/1
  Demux3/6 -> Product18/2
  Demux3/5 -> Product17/2
  Demux3/4 -> Product16/2
  Demux3/3 -> Product15/2
  Demux3/2 -> Product14/2
  Demux3/1 -> Product13/2
  Constant5/1 -> Product1/1
  Constant1/1 -> Product2/1
  Constant2/1 -> Product3/1
  Constant3/1 -> Product25/1
  Constant4/1 -> Product26/1
  Constant6/1 -> Product27/1
  Constant7/1 -> Product40/1
  Constant8/1 -> Product11/1
  Constant9/1 -> Product18/1
  Demux1/1 -> Subsystem5/2(In2), Subsystem15/2(In2), Subsystem15/3(In3), Subsystem20/2(In2), Subsystem20/3(In3), Subsystem7/3(In3), Subsystem7/2(In2), Subsystem5/3(In3)
  Demux1/2 -> Subsystem11/3(In3), Subsystem19/2(In2), Subsystem19/3(In3), Subsystem11/2(In2), Subsystem6/3(In3), Subsystem6/2(In2), Subsystem2/3(In3), Subsystem2/2(In2)
  Demux1/3 -> Subsystem3/2(In2), Subsystem3/3(In3), Subsystem10/2(In2), Subsystem10/3(In3), Subsystem14/2(In2), Subsystem14/3(In3), Subsystem1/3(In3), Subsystem1/2(In2)
  Subsystem/1(Out1) -> Product34/1
  Subsystem1/1(Out1) -> Product35/1
  Subsystem2/1(Out1) -> Product36/1
  Add6/1 -> Mux/1
  Subsystem3/1(Out1) -> Product4/1
  Subsystem4/1(Out1) -> Product5/1
  Subsystem5/1(Out1) -> Product6/1
  Add1/1 -> Mux/2
  Subsystem6/1(Out1) -> Product28/1
  Subsystem7/1(Out1) -> Product29/1
  Subsystem8/1(Out1) -> Product30/1
  Add5/1 -> Mux/3
  Subsystem9/1(Out1) -> Product37/1
  Subsystem10/1(Out1) -> Product38/1
  Subsystem11/1(Out1) -> Product39/1
  Subsystem12/1(Out1) -> Product41/1
  Subsystem13/1(Out1) -> Product42/1
  Add7/1 -> Mux/4
  Subsystem14/1(Out1) -> Product7/1
  Demux1/4 -> Subsystem3/1(In1), Subsystem4/2(In2), Subsystem8/1(In1), Subsystem10/1(In1), Subsystem11/1(In1), Subsystem12/2(In2), Subsystem13/2(In2), Subsystem16/2(In2), Subsystem17/2(In2), Subsystem18/3(In3), Subsystem18/4(In4), Subsystem21/1(In1), Subsystem22/2(In2), Subsystem23/3(In3), Subsystem23/4(In4), Subsystem6/1(In1)
  Subsystem16/1(Out1) -> Product8/1
  Subsystem15/1(Out1) -> Product9/1
  Demux1/6 -> Subsystem4/1(In1), Subsystem5/1(In1), Subsystem12/4(In4), Subsystem13/1(In1), Subsystem16/1(In1), Subsystem17/4(In4), Subsystem18/1(In1), Subsystem19/1(In1), Subsystem20/1(In1), Subsystem22/1(In1), Subsystem23/1(In1), Subsystem17/3(In3), Subsystem12/3(In3), Subsystem9/2(In2), Subsystem2/1(In1), Subsystem/1(In1)
  Subsystem17/1(Out1) -> Product10/1
  Subsystem18/1(Out1) -> Product12/1
  Subsystem19/1(Out1) -> Product13/1
  Add2/1 -> Mux/5
  Subsystem20/1(Out1) -> Product14/1
  Subsystem21/1(Out1) -> Product15/1
  Demux1/5 -> Subsystem12/1(In1), Subsystem13/3(In3), Subsystem13/4(In4), Subsystem15/1(In1), Subsystem17/1(In1), Subsystem18/2(In2), Subsystem21/2(In2), Subsystem22/4(In4), Subsystem23/2(In2), Subsystem22/3(In3), Subsystem14/1(In1), Subsystem9/1(In1), Subsystem8/2(In2), Subsystem7/1(In1), Subsystem1/1(In1), Subsystem/2(In2)
  Subsystem22/1(Out1) -> Product16/1
  Subsystem23/1(Out1) -> Product17/1
  Add3/1 -> Mux/6

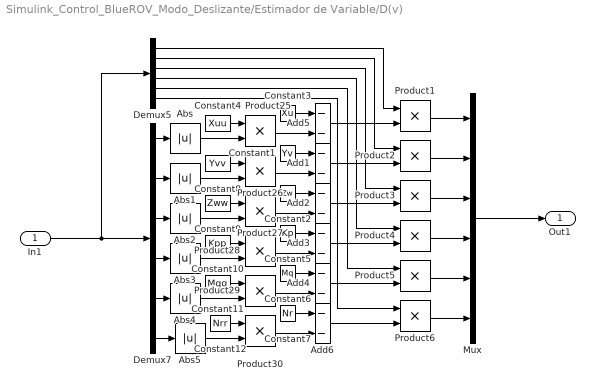
== system Simulink_Control_BlueROV_Modo_Deslizante/Estimador de Variable/D(v) ==
  In1 : Inport
  Abs{,1..5} (6 alike) : Abs
  Add{1..6} (6 alike) : Sum  Inputs=--
  Constant1 : Constant  Value=Yv
  Constant10 : Constant  Value=Kpp
  Constant11 : Constant  Value=Mqq
  Constant12 : Constant  Value=Nrr
  Constant2 : Constant  Value=Zw
  Constant3 : Constant  Value=Xu
  Constant4 : Constant  Value=Xuu
  Constant5 : Constant  Value=Kp
  Constant6 : Constant  Value=Mq
  Constant7 : Constant  Value=Nr
  Constant8 : Constant  Value=Yvv
  Constant9 : Constant  Value=Zww
  Demux5 : Demux  Outputs=6
  Demux7 : Demux  Outputs=6
  Mux : Mux  Inputs=6
  Product{1..6,25..30} (12 alike) : Product
  Out1 : Outport
  wires:
  In1/1 -> Demux5/1, Demux7/1
  ? -> ?
  ? -> ?
  Mux/1 -> Out1/1
  Abs/1 -> Product25/2
  Demux7/2 -> Abs1/1
  Abs1/1 -> Product26/2
  Demux7/1 -> Abs/1
  Demux7/3 -> Abs2/1
  Abs2/1 -> Product27/2
  Demux7/4 -> Abs3/1
  Abs3/1 -> Product28/2
  Abs4/1 -> Product29/2
  Demux7/5 -> Abs4/1
  Abs5/1 -> Product30/2
  Demux7/6 -> Abs5/1
  Product25/1 -> Add5/2
  Product26/1 -> Add1/2
  Product27/1 -> Add2/2
  Product28/1 -> Add3/2
  Product29/1 -> Add4/2
  Product30/1 -> Add6/2
  Product6/1 -> Mux/6
  Product5/1 -> Mux/5
  Product4/1 -> Mux/4
  Product3/1 -> Mux/3
  Product2/1 -> Mux/2
  Product1/1 -> Mux/1
  Add6/1 -> Product6/2
  Add4/1 -> Product5/2
  Add3/1 -> Product4/2
  Add2/1 -> Product3/2
  Add1/1 -> Product2/2
  Add5/1 -> Product1/2
  Demux5/6 -> Product6/1
  Demux5/5 -> Product5/1
  Demux5/4 -> Product4/1
  Demux5/3 -> Product3/1
  Demux5/2 -> Product2/1
  Demux5/1 -> Product1/1
  Constant1/1 -> Add1/1
  Constant2/1 -> Add2/1
  Constant3/1 -> Add5/1
  Constant5/1 -> Add3/1
  Constant6/1 -> Add4/1
  Constant7/1 -> Add6/1
  Constant4/1 -> Product25/1
  Constant8/1 -> Product26/1
  Constant12/1 -> Product30/1
  Constant11/1 -> Product29/1
  Constant10/1 -> Product28/1
  Constant9/1 -> Product27/1

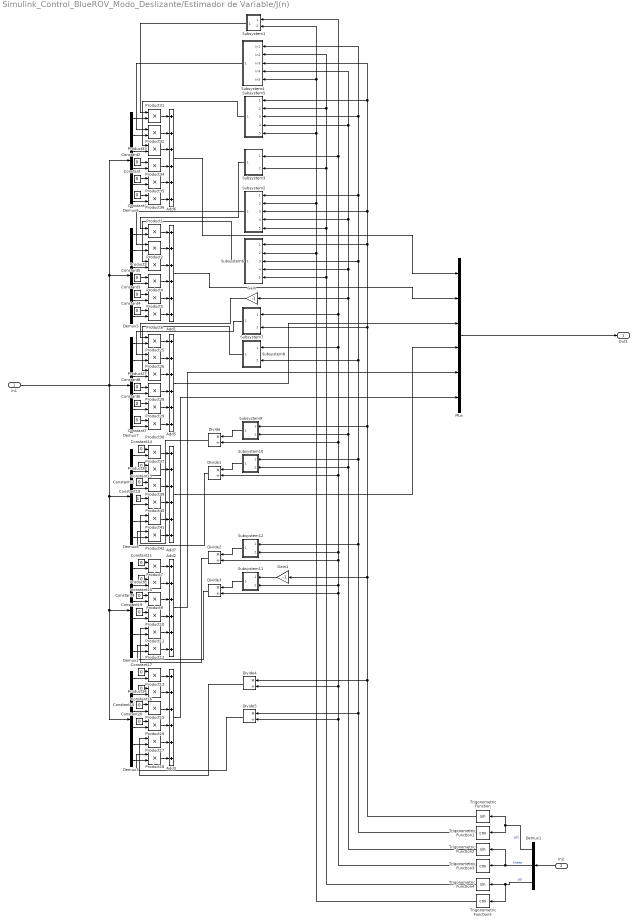
== system Simulink_Control_BlueROV_Modo_Deslizante/Estimador de Variable/J(n) ==
  In1 : Inport
  In2 : Inport  Port=2
  Add{1..3,5..7} (6 alike) : Sum  Inputs=++++++
  Constant{,1..17,19..20} (20 alike) : Constant  Value=0
  Constant18 : Constant
  Demux1 : Demux  Outputs=3
  Demux{2..3,5..8} (6 alike) : Demux  Outputs=6
  Divide{,1..5} (6 alike) : Product  Inputs=*/
  Gain : Gain  Gain=-1
  Gain1 : Gain  Gain=-1
  Mux : Mux  Inputs=6
  Product{1..18,25..42} (36 alike) : Product
  Subsystem1 : Subsystem
  Subsystem10 : Subsystem
  Subsystem11 : Subsystem
  Subsystem12 : Subsystem
  Subsystem2 : Subsystem
  Subsystem3 : Subsystem
  Subsystem4 : Subsystem
  Subsystem5 : Subsystem
  Subsystem6 : Subsystem
  Subsystem7 : Subsystem
  Subsystem8 : Subsystem
  Subsystem9 : Subsystem
  Trigonometric Function : Trigonometry
  Trigonometric Function1 : Trigonometry  Operator=cos
  Trigonometric Function2 : Trigonometry
  Trigonometric Function3 : Trigonometry  Operator=cos
  Trigonometric Function4 : Trigonometry
  Trigonometric Function5 : Trigonometry  Operator=cos
  Out1 : Outport
  wires:
  Divide5/1 -> Product18/1
  Divide3/1 -> Product12/1
  Subsystem1/1(Out1) -> Product31/1
  Constant12/1 -> Product39/1
  Subsystem5/1(Out1) -> Product33/1
  Constant13/1 -> Product38/1
  Subsystem10/1(Out1) -> Divide1/1
  Divide1/1 -> Product42/1
  Demux7/3 -> Product27/2
  Product28/1 -> Add5/4
  Product29/1 -> Add5/5
  Product25/1 -> Add5/1
  Product30/1 -> Add5/6
  Demux7/6 -> Product30/2
  Constant8/1 -> Product28/1
  Demux7/1 -> Product25/2
  Demux7/4 -> Product28/2
  Product27/1 -> Add5/3
  Constant6/1 -> Product29/1
  Product11/1 -> Add2/5
  Demux2/3 -> Product9/2
  Product7/1 -> Add2/1
  Demux2/1 -> Product7/2
  Demux2/5 -> Product11/2
  Demux2/4 -> Product10/2
  Product9/1 -> Add2/3
  Demux2/2 -> Product8/2
  Constant10/1 -> Product8/1
  Trigonometric Function3/1 -> Divide5/2, Divide4/2, Divide3/2, Subsystem11/2(In2), Divide2/2, Subsystem12/2(In2), Divide1/2, Divide/2, Subsystem8/1(In1), Subsystem7/1(In1), Subsystem3/1(In1), Subsystem1/1(In1)
  Demux8/2 -> Product38/2
  Product39/1 -> Add7/3
  Product38/1 -> Add7/2
  In1/1 -> Demux5/1, Demux6/1, Demux7/1, Demux8/1, Demux3/1, Demux2/1
  Subsystem9/1(Out1) -> Divide/1
  Add2/1 -> Mux/5
  Subsystem11/1(Out1) -> Divide3/1
  Product10/1 -> Add2/4
  Subsystem12/1(Out1) -> Divide2/1
  Constant19/1 -> Product10/1
  Trigonometric Function1/1 -> Divide5/1, Subsystem10/1(In1), Subsystem8/2(In2), Subsystem6/3(In3), Subsystem2/1(In1), Subsystem5/3(In3), Subsystem4/1(In1), Subsystem12/1(In1)
  Add1/1 -> Mux/2
  Mux/1 -> Out1/1
  Add6/1 -> Mux/1
  Add3/1 -> Mux/6
  Product12/1 -> Add2/6
  Add7/1 -> Mux/4
  Divide4/1 -> Product17/1
  Add5/1 -> Mux/3
  Product26/1 -> Add5/2
  Constant7/1 -> Product30/1
  Trigonometric Function/1 -> Divide4/1, Gain1/1, Subsystem9/1(In1), Subsystem7/2(In2), Subsystem6/1(In1), Subsystem2/3(In3), Subsystem5/1(In1), Subsystem4/3(In3)
  Constant14/1 -> Product37/1
  Gain/1 -> Product25/1
  Trigonometric Function5/1 -> Subsystem6/2(In2), Subsystem5/5(In5), Subsystem4/5(In5), Subsystem1/2(In2), Subsystem2/2(In2)
  Subsystem8/1(Out1) -> Product27/1
  Subsystem3/1(Out1) -> Product1/1
  Subsystem6/1(Out1) -> Product3/1
  Demux7/2 -> Product26/2
  Constant20/1 -> Product16/1
  Subsystem7/1(Out1) -> Product26/1
  Demux7/5 -> Product29/2
  Constant15/1 -> Product15/1
  Constant16/1 -> Product14/1
  Demux3/2 -> Product14/2
  Product15/1 -> Add3/3
  Constant17/1 -> Product13/1
  Product14/1 -> Add3/2
  Constant11/1 -> Product7/1
  Trigonometric Function4/1 -> Subsystem6/5(In5), Subsystem2/5(In5), Subsystem3/2(In2), Subsystem5/2(In2), Subsystem4/2(In2)
  Subsystem4/1(Out1) -> Product32/1
  Product13/1 -> Add3/1
  Product16/1 -> Add3/4
  Demux3/1 -> Product13/2
  Demux3/4 -> Product16/2
  Demux3/3 -> Product15/2
  Trigonometric Function2/1 -> Subsystem10/2(In2), Subsystem9/2(In2), Gain/1, Subsystem6/4(In4), Subsystem2/4(In4), Subsystem5/4(In4), Subsystem4/4(In4)
  Constant1/1 -> Product36/1
  Product17/1 -> Add3/5
  Demux5/3 -> Product3/2
  Product6/1 -> Add1/6
  Demux5/5 -> Product5/2
  Demux5/4 -> Product4/2
  Demux5/1 -> Product1/2
  Demux1/1 -> Trigonometric Function/1, Trigonometric Function1/1  "phi"
  Constant4/1 -> Product6/1
  Constant2/1 -> Product34/1
  Constant/1 -> Product35/1
  Demux8/6 -> Product42/2
  Demux3/5 -> Product17/2
  Product4/1 -> Add1/4
  Constant18/1 -> Product40/1
  Product37/1 -> Add7/1
  Demux2/6 -> Product12/2
  Demux8/4 -> Product40/2
  Gain1/1 -> Subsystem11/1(In1)
  Product42/1 -> Add7/6
  Constant3/1 -> Product5/1
  Product8/1 -> Add2/2
  Demux8/5 -> Product41/2
  Product1/1 -> Add1/1
  Demux8/3 -> Product39/2
  Product3/1 -> Add1/3
  Divide2/1 -> Product11/1
  Product18/1 -> Add3/6
  Demux1/3 -> Trigonometric Function5/1, Trigonometric Function4/1  "psi"
  Constant5/1 -> Product4/1
  Demux5/2 -> Product2/2
  Divide/1 -> Product41/1
  Product32/1 -> Add6/2
  Product2/1 -> Add1/2
  Product34/1 -> Add6/4
  Demux6/1 -> Product31/2
  Demux6/6 -> Product36/2
  Product41/1 -> Add7/5
  Demux6/5 -> Product35/2
  Product5/1 -> Add1/5
  Constant9/1 -> Product9/1
  Demux3/6 -> Product18/2
  Product33/1 -> Add6/3
  Demux1/2 -> Trigonometric Function2/1, Trigonometric Function3/1  "theta"
  Demux6/4 -> Product34/2
  Demux6/3 -> Product33/2
  Demux5/6 -> Product6/2
  Product36/1 -> Add6/6
  Demux6/2 -> Product32/2
  Subsystem2/1(Out1) -> Product2/1
  Product40/1 -> Add7/4
  Demux8/1 -> Product37/2
  Product31/1 -> Add6/1
  Product35/1 -> Add6/5
  In2/1 -> Demux1/1

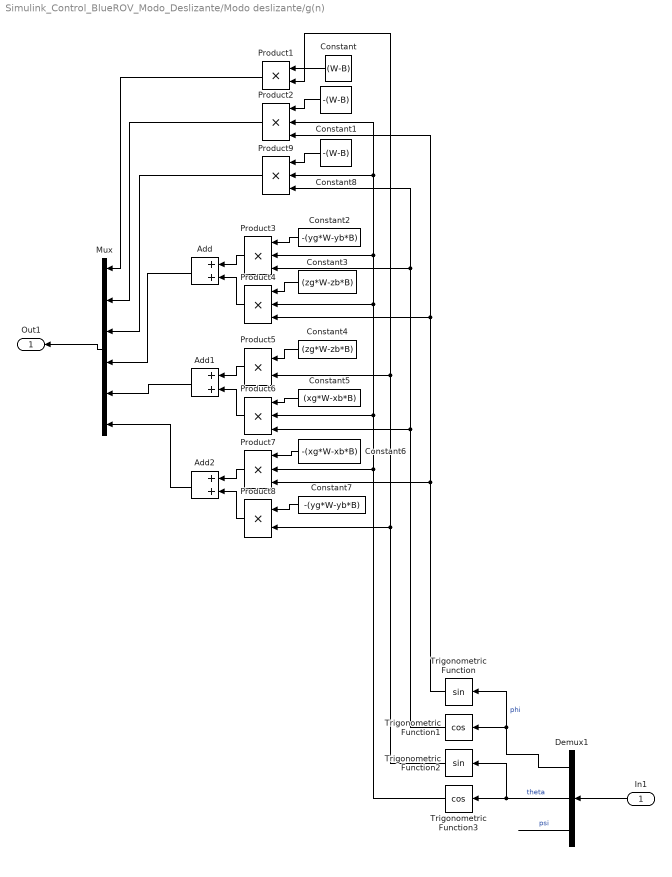
== system Simulink_Control_BlueROV_Modo_Deslizante/Modo deslizante/g(n) ==
  In1 : Inport
  Add : Sum
  Add1 : Sum
  Add2 : Sum
  Constant : Constant  Value=(W-B)
  Constant1 : Constant  Value=-(W-B)
  Constant2 : Constant  Value=-(yg*W-yb*B)
  Constant3 : Constant  Value=(zg*W-zb*B)
  Constant4 : Constant  Value=(zg*W-zb*B)
  Constant5 : Constant  Value=(xg*W-xb*B)
  Constant6 : Constant  Value=-(xg*W-xb*B)
  Constant7 : Constant  Value=-(yg*W-yb*B)
  Constant8 : Constant  Value=-(W-B)
  Demux1 : Demux  Outputs=3
  Mux : Mux  Inputs=6
  Product1 : Product
  Product{2..4,6..7,9} (6 alike) : Product  Inputs=3
  Product5 : Product
  Product8 : Product
  Trigonometric Function : Trigonometry
  Trigonometric Function1 : Trigonometry  Operator=cos
  Trigonometric Function2 : Trigonometry
  Trigonometric Function3 : Trigonometry  Operator=cos
  Out1 : Outport
  wires:
  Demux1/3 -> ?  "psi"
  Demux1/1 -> Trigonometric Function/1, Trigonometric Function1/1  "phi"
  Demux1/2 -> Trigonometric Function2/1, Trigonometric Function3/1  "theta"
  In1/1 -> Demux1/1
  Mux/1 -> Out1/1
  Product1/1 -> Mux/1
  Constant/1 -> Product1/1
  Trigonometric Function2/1 -> Product8/2, Product5/2, Product1/2
  Constant1/1 -> Product2/1
  Trigonometric Function/1 -> Product7/3, Product4/3, Product2/3
  Product2/1 -> Mux/2
  Product7/1 -> Add2/1
  Product8/1 -> Add2/2
  Product6/1 -> Add1/2
  Constant5/1 -> Product6/1
  Constant2/1 -> Product3/1
  Constant4/1 -> Product5/1
  Product4/1 -> Add/2
  Constant3/1 -> Product4/1
  Product3/1 -> Add/1
  Product5/1 -> Add1/1
  Constant7/1 -> Product8/1
  Constant8/1 -> Product9/1
  Product9/1 -> Mux/3
  Add/1 -> Mux/4
  Add1/1 -> Mux/5
  Constant6/1 -> Product7/1
  Add2/1 -> Mux/6
  Trigonometric Function1/1 -> Product6/3, Product3/3, Product9/3
  Trigonometric Function3/1 -> Product7/2, Product6/2, Product4/2, Product3/2, Product9/2, Product2/2

== system Simulink_Control_BlueROV_Modo_Deslizante/BlueRov2/C(v)/Subsystem ==
  In1 : Inport
  In2 : Inport  Port=2
  Add4 : Sum
  Constant : Constant  Value=zg
  Constant10 : Constant  Value=yg
  Gain : Gain  Gain=m
  Product19 : Product
  Product20 : Product
  Out1 : Outport
  wires:
  Product20/1 -> Add4/2
  Product19/1 -> Add4/1
  In1/1 -> Product19/2
  Constant/1 -> Product19/1
  Gain/1 -> Out1/1
  Constant10/1 -> Product20/1
  Add4/1 -> Gain/1
  In2/1 -> Product20/2

== system Simulink_Control_BlueROV_Modo_Deslizante/BlueRov2/C(v)/Subsystem1 ==
  In1 : Inport
  In2 : Inport  Port=2
  In3 : Inport  Port=3
  Add4 : Sum  Inputs=+-
  Add8 : Sum  Inputs=-+
  Constant : Constant  Value=xg
  Constant10 : Constant
  Constant11 : Constant  Value=-Zwdot
  Gain : Gain  Gain=m
  Product19 : Product
  Product20 : Product
  Product21 : Product
  Out1 : Outport
  wires:
  Product20/1 -> Add4/2
  Constant11/1 -> Product21/1
  Gain/1 -> Add8/1
  Product19/1 -> Add4/1
  Constant/1 -> Product19/1
  Product21/1 -> Add8/2
  Add4/1 -> Gain/1
  Constant10/1 -> Product20/1
  Add8/1 -> Out1/1
  In1/1 -> Product19/2
  In3/1 -> Product21/2
  In2/1 -> Product20/2

== system Simulink_Control_BlueROV_Modo_Deslizante/BlueRov2/C(v)/Subsystem10 ==
  In1 : Inport
  In2 : Inport  Port=2
  In3 : Inport  Port=3
  Add4 : Sum
  Add8 : Sum
  Constant : Constant  Value=yg
  Constant10 : Constant
  Constant11 : Constant  Value=-Zwdot
  Gain : Gain  Gain=m
  Product19 : Product
  Product20 : Product
  Product21 : Product
  Out1 : Outport
  wires:
  In2/1 -> Product20/2
  In3/1 -> Product21/2
  In1/1 -> Product19/2
  Add8/1 -> Out1/1
  Constant10/1 -> Product20/1
  Add4/1 -> Gain/1
  Product21/1 -> Add8/2
  Constant/1 -> Product19/1
  Product19/1 -> Add4/1
  Gain/1 -> Add8/1
  Constant11/1 -> Product21/1
  Product20/1 -> Add4/2

== system Simulink_Control_BlueROV_Modo_Deslizante/BlueRov2/C(v)/Subsystem11 ==
  In1 : Inport
  In2 : Inport  Port=2
  In3 : Inport  Port=3
  Add4 : Sum  Inputs=+-
  Add8 : Sum
  Constant : Constant  Value=zg
  Constant10 : Constant
  Constant11 : Constant  Value=Yvdot
  Gain : Gain  Gain=m
  Product19 : Product
  Product20 : Product
  Product21 : Product
  Out1 : Outport
  wires:
  Product20/1 -> Add4/2
  Constant11/1 -> Product21/1
  Gain/1 -> Add8/1
  Product19/1 -> Add4/1
  Constant/1 -> Product19/1
  Product21/1 -> Add8/2
  Add4/1 -> Gain/1
  Constant10/1 -> Product20/1
  Add8/1 -> Out1/1
  In1/1 -> Product19/2
  In3/1 -> Product21/2
  In2/1 -> Product20/2

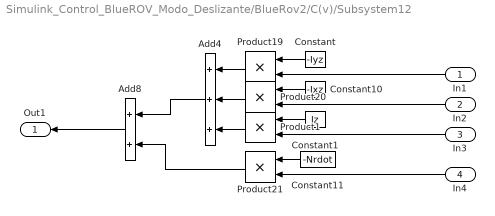
== system Simulink_Control_BlueROV_Modo_Deslizante/BlueRov2/C(v)/Subsystem12 ==
  In1 : Inport
  In2 : Inport  Port=2
  In3 : Inport  Port=3
  In4 : Inport  Port=4
  Add4 : Sum  Inputs=+++
  Add8 : Sum
  Constant : Constant  Value=-Iyz
  Constant1 : Constant  Value=Iz
  Constant10 : Constant  Value=-Ixz
  Constant11 : Constant  Value=-Nrdot
  Product{1,19..21} (4 alike) : Product
  Out1 : Outport
  wires:
  In2/1 -> Product20/2
  In1/1 -> Product19/2
  Add8/1 -> Out1/1
  Constant10/1 -> Product20/1
  Product21/1 -> Add8/2
  Constant/1 -> Product19/1
  Product19/1 -> Add4/1
  Add4/1 -> Add8/1
  Constant11/1 -> Product21/1
  Product20/1 -> Add4/2
  Product1/1 -> Add4/3
  Constant1/1 -> Product1/1
  In4/1 -> Product21/2
  In3/1 -> Product1/2

== system Simulink_Control_BlueROV_Modo_Deslizante/BlueRov2/C(v)/Subsystem13 ==
  In1 : Inport
  In2 : Inport  Port=2
  In3 : Inport  Port=3
  In4 : Inport  Port=4
  Add4 : Sum  Inputs=+++
  Add8 : Sum
  Constant : Constant  Value=Iyz
  Constant1 : Constant  Value=-Iy
  Constant10 : Constant  Value=Ixy
  Constant11 : Constant  Value=Mqdot
  Product{1,19..21} (4 alike) : Product
  Out1 : Outport
  wires:
  In3/1 -> Product1/2
  In4/1 -> Product21/2
  Constant1/1 -> Product1/1
  Product1/1 -> Add4/3
  Product20/1 -> Add4/2
  Constant11/1 -> Product21/1
  Add4/1 -> Add8/1
  Product19/1 -> Add4/1
  Constant/1 -> Product19/1
  Product21/1 -> Add8/2
  Constant10/1 -> Product20/1
  Add8/1 -> Out1/1
  In1/1 -> Product19/2
  In2/1 -> Product20/2

== system Simulink_Control_BlueROV_Modo_Deslizante/BlueRov2/C(v)/Subsystem14 ==
  In1 : Inport
  In2 : Inport  Port=2
  In3 : Inport  Port=3
  Add4 : Sum  Inputs=+-
  Add8 : Sum
  Constant : Constant  Value=xg
  Constant10 : Constant
  Constant11 : Constant  Value=Zwdot
  Gain : Gain  Gain=m
  Product19 : Product
  Product20 : Product
  Product21 : Product
  Out1 : Outport
  wires:
  Product20/1 -> Add4/2
  Constant11/1 -> Product21/1
  Gain/1 -> Add8/1
  Product19/1 -> Add4/1
  Constant/1 -> Product19/1
  Product21/1 -> Add8/2
  Add4/1 -> Gain/1
  Constant10/1 -> Product20/1
  Add8/1 -> Out1/1
  In1/1 -> Product19/2
  In3/1 -> Product21/2
  In2/1 -> Product20/2

== system Simulink_Control_BlueROV_Modo_Deslizante/BlueRov2/C(v)/Subsystem15 ==
  In1 : Inport
  In2 : Inport  Port=2
  In3 : Inport  Port=3
  Add4 : Sum
  Add8 : Sum
  Constant : Constant  Value=zg
  Constant10 : Constant
  Constant11 : Constant  Value=-Xudot
  Gain : Gain  Gain=m
  Product19 : Product
  Product20 : Product
  Product21 : Product
  Out1 : Outport
  wires:
  In2/1 -> Product20/2
  In3/1 -> Product21/2
  In1/1 -> Product19/2
  Add8/1 -> Out1/1
  Constant10/1 -> Product20/1
  Add4/1 -> Gain/1
  Product21/1 -> Add8/2
  Constant/1 -> Product19/1
  Product19/1 -> Add4/1
  Gain/1 -> Add8/1
  Constant11/1 -> Product21/1
  Product20/1 -> Add4/2

== system Simulink_Control_BlueROV_Modo_Deslizante/BlueRov2/C(v)/Subsystem16 ==
  In1 : Inport
  In2 : Inport  Port=2
  Add4 : Sum
  Constant : Constant  Value=zg
  Constant10 : Constant  Value=xg
  Gain : Gain  Gain=-m
  Product19 : Product
  Product20 : Product
  Out1 : Outport
  wires:
  Product20/1 -> Add4/2
  Product19/1 -> Add4/1
  In1/1 -> Product19/2
  Constant/1 -> Product19/1
  Gain/1 -> Out1/1
  Constant10/1 -> Product20/1
  Add4/1 -> Gain/1
  In2/1 -> Product20/2

== system Simulink_Control_BlueROV_Modo_Deslizante/BlueRov2/C(v)/Subsystem17 ==
  In1 : Inport
  In2 : Inport  Port=2
  In3 : Inport  Port=3
  In4 : Inport  Port=4
  Add4 : Sum  Inputs=+++
  Add8 : Sum
  Constant : Constant  Value=Iyz
  Constant1 : Constant  Value=-Iz
  Constant10 : Constant  Value=Ixz
  Constant11 : Constant  Value=Nrdot
  Product{1,19..21} (4 alike) : Product
  Out1 : Outport
  wires:
  In3/1 -> Product1/2
  In4/1 -> Product21/2
  Constant1/1 -> Product1/1
  Product1/1 -> Add4/3
  Product20/1 -> Add4/2
  Constant11/1 -> Product21/1
  Add4/1 -> Add8/1
  Product19/1 -> Add4/1
  Constant/1 -> Product19/1
  Product21/1 -> Add8/2
  Constant10/1 -> Product20/1
  Add8/1 -> Out1/1
  In1/1 -> Product19/2
  In2/1 -> Product20/2

== system Simulink_Control_BlueROV_Modo_Deslizante/BlueRov2/C(v)/Subsystem18 ==
  In1 : Inport
  In2 : Inport  Port=2
  In3 : Inport  Port=3
  In4 : Inport  Port=4
  Add4 : Sum  Inputs=+++
  Add8 : Sum
  Constant : Constant  Value=-Ixz
  Constant1 : Constant  Value=Ix
  Constant10 : Constant  Value=-Ixy
  Constant11 : Constant  Value=-Kpdot
  Product{1,19..21} (4 alike) : Product
  Out1 : Outport
  wires:
  In2/1 -> Product20/2
  In1/1 -> Product19/2
  Add8/1 -> Out1/1
  Constant10/1 -> Product20/1
  Product21/1 -> Add8/2
  Constant/1 -> Product19/1
  Product19/1 -> Add4/1
  Add4/1 -> Add8/1
  Constant11/1 -> Product21/1
  Product20/1 -> Add4/2
  Product1/1 -> Add4/3
  Constant1/1 -> Product1/1
  In4/1 -> Product21/2
  In3/1 -> Product1/2

== system Simulink_Control_BlueROV_Modo_Deslizante/BlueRov2/C(v)/Subsystem19 ==
  In1 : Inport
  In2 : Inport  Port=2
  In3 : Inport  Port=3
  Add4 : Sum
  Add8 : Sum
  Constant : Constant  Value=xg
  Constant10 : Constant
  Constant11 : Constant  Value=-Yvdot
  Gain : Gain  Gain=m
  Product19 : Product
  Product20 : Product
  Product21 : Product
  Out1 : Outport
  wires:
  In2/1 -> Product20/2
  In3/1 -> Product21/2
  In1/1 -> Product19/2
  Add8/1 -> Out1/1
  Constant10/1 -> Product20/1
  Add4/1 -> Gain/1
  Product21/1 -> Add8/2
  Constant/1 -> Product19/1
  Product19/1 -> Add4/1
  Gain/1 -> Add8/1
  Constant11/1 -> Product21/1
  Product20/1 -> Add4/2

== system Simulink_Control_BlueROV_Modo_Deslizante/BlueRov2/C(v)/Subsystem2 ==
  In1 : Inport
  In2 : Inport  Port=2
  In3 : Inport  Port=3
  Add10 : Sum  Inputs=-+
  Add9 : Sum
  Constant12 : Constant  Value=xg
  Constant13 : Constant
  Constant14 : Constant  Value=Yvdot
  Gain1 : Gain  Gain=m
  Product22 : Product
  Product23 : Product
  Product24 : Product
  Out1 : Outport
  wires:
  In1/1 -> Product22/2
  Constant14/1 -> Product24/1
  Add9/1 -> Gain1/1
  Constant12/1 -> Product22/1
  Product23/1 -> Add9/2
  Gain1/1 -> Add10/1
  Constant13/1 -> Product23/1
  Product24/1 -> Add10/2
  Product22/1 -> Add9/1
  In3/1 -> Product24/2
  Add10/1 -> Out1/1
  In2/1 -> Product23/2

== system Simulink_Control_BlueROV_Modo_Deslizante/BlueRov2/C(v)/Subsystem20 ==
  In1 : Inport
  In2 : Inport  Port=2
  In3 : Inport  Port=3
  Add4 : Sum
  Add8 : Sum
  Constant : Constant  Value=yg
  Constant10 : Constant  Value=-1
  Constant11 : Constant  Value=Xudot
  Gain : Gain  Gain=m
  Product19 : Product
  Product20 : Product
  Product21 : Product
  Out1 : Outport
  wires:
  Product20/1 -> Add4/2
  Constant11/1 -> Product21/1
  Gain/1 -> Add8/1
  Product19/1 -> Add4/1
  Constant/1 -> Product19/1
  Product21/1 -> Add8/2
  Add4/1 -> Gain/1
  Constant10/1 -> Product20/1
  Add8/1 -> Out1/1
  In1/1 -> Product19/2
  In3/1 -> Product21/2
  In2/1 -> Product20/2

== system Simulink_Control_BlueROV_Modo_Deslizante/BlueRov2/C(v)/Subsystem21 ==
  In1 : Inport
  In2 : Inport  Port=2
  Add4 : Sum
  Constant : Constant  Value=xg
  Constant10 : Constant  Value=yg
  Gain : Gain  Gain=-m
  Product19 : Product
  Product20 : Product
  Out1 : Outport
  wires:
  In2/1 -> Product20/2
  Add4/1 -> Gain/1
  Constant10/1 -> Product20/1
  Gain/1 -> Out1/1
  Constant/1 -> Product19/1
  In1/1 -> Product19/2
  Product19/1 -> Add4/1
  Product20/1 -> Add4/2
